simulink model "click_transpose"  (Simulink 10.0)
settings: Solver=VariableStepAuto  StartTime=0.0  StopTime=4  RelTol=1e-3
undefined symbols (not defined in the file or in its folder): DiscIntNeverNeededParam, q0, Tc
settings Model: LogicAnalyzerSignalOrdering=de64767a-5a6d-4200-a971-f55b6b3f8a08  Creator=swl782203812  LastModifiedBy=swl782203812
settings DataIOCC: SaveFormat=Dataset  ReturnWorkspaceOutputs=on
settings OptimizationCC: LifeSpan=auto
settings DebuggingCC: UnderspecifiedInitializationDetection=Simplified  MergeDetectMultiDrivingBlocksExec=error  SFUnexpectedBacktrackingDiag=error  SFNoUnconditionalDefaultTransitionDiag=error  SFExecutionAtInitializationDiag=warning
settings HardwareCC: ProdBitPerPointer=64  ProdBitPerSizeT=64  ProdBitPerPtrDiffT=64  ProdLargestAtomicFloat=Float  ProdIntDivRoundTo=Zero  ProdEndianess=LittleEndian  ProdWordSize=64  ProdHWDeviceType=Intel->x86-64 (Windows64)
settings ModelReferenceCC: PropagateSignalLabelsOutOfModel=on
settings SFSimCC: SimUseLocalCustomCode=on
settings RTWCC: RTWUseLocalCustomCode=on
settings CodeAppCC: StateflowObjectComments=off
settings GRTTargetCC: TargetLangStandard=C99 (ISO)  CombineOutputUpdateFcns=on  GRTInterface=off
settings ConfigComp: CovMetricSettings=dwe  CovHtmlReporting=off  CovSaveCumulativeToWorkspaceVar=off  CovSaveSingleToWorkspaceVar=off

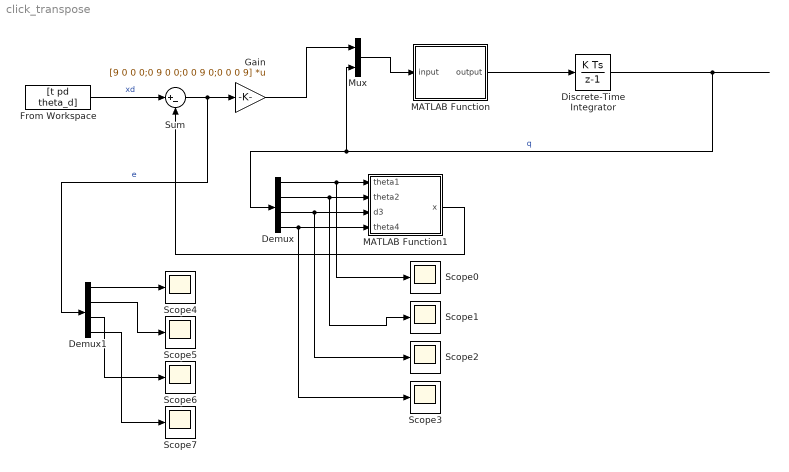
== system click_transpose ==
  Demux : Demux
  Demux1 : Demux
  Discrete-Time Integrator : DiscreteIntegrator  InitialCondition=q0  SampleTime=Tc  ICPrevOutput=DiscIntNeverNeededParam  ICPrevScaledInput=DiscIntNeverNeededParam
  From Workspace : FromWorkspace  VariableName=[t pd theta_d]  SampleTime=Tc
  Gain : Gain  Gain=[9 0 0 0;0 9 0 0;0 0 9 0;0 0 0 9]  Multiplication=Matrix(K*u) (u vector)
  MATLAB Function : MATLAB Function  TreatAsAtomicUnit=on
  MATLAB Function1 : MATLAB Function  TreatAsAtomicUnit=on
  Mux : Mux  Inputs=2
  Scope{0..7} (8 alike) : Scope
  Sum : Sum  Inputs=|+-
  wires:
  From Workspace/1 -> Sum/1  "xd"
  Sum/1 -> Demux1/1, Gain/1  "e"
  Discrete-Time Integrator/1 -> Mux/2, Demux/1  "q"
  Gain/1 -> Mux/1
  MATLAB Function1/1(x) -> Sum/2
  Demux/1 -> Scope0/1, MATLAB Function1/1(theta1)
  Demux/2 -> Scope1/1, MATLAB Function1/2(theta2)
  Demux/3 -> Scope2/1, MATLAB Function1/3(d3)
  Demux/4 -> Scope3/1, MATLAB Function1/4(theta4)
  MATLAB Function/1(output) -> Discrete-Time Integrator/1
  Mux/1 -> MATLAB Function/1(input)
  Demux1/1 -> Scope4/1
  Demux1/2 -> Scope5/1
  Demux1/3 -> Scope6/1
  Demux1/4 -> Scope7/1

== matlab function MATLAB Function ==
  data: input input double; output output double
function output=Jacobian_tranpose(input)
%INPUT is (theta1, theta2, d3, theta4,xd_dot_plus_Ke) 
theta1=input(5,:); d1=0; a1=0.5; alpha1=0; %parameter link1
theta2=input(6,:); d2=0; a2=0.5; alpha2=0; %parameter link2
theta3=0; d3=input(7,:); a3=0; alpha3=0;  %parameter link3
theta4=input(8,:); d4=0; a4=0; alpha4=0;  %parameter link4
 T01=DHmatrix(theta1,d1,a1,alpha1);
 T12=DHmatrix(theta2,d2,a2,alpha2);
 T23=DHmatrix(theta3,d3,a3,alpha3);
 T34=DHmatrix(theta4,d4,a4,alpha4);
 T02=T01*T12;
 T03=T01*T12*T23;
 T04=T01*T12*T23*T34;
P0=[0;0;0];
P1=T01(1:3,4);
P3=T03(1:3,4);
P4=T04(1:3,4);

Z0=[0;0;1];
Jv1=cross(Z0,(P4-P0));
Jv2=cross(Z0,(P4-P1));
Jv3=Z0;
Jv4=cross(Z0,(P4-P3));
Jv=[Jv1 Jv2 Jv3 Jv4;1 1 0 1];
output=Jv'*input(1:4,:);
end

function [Mdh] = DHmatrix(theta,d,a,alpha)
%DHMATRIX Summary of this function goes here
%   inputannya DH parameter
Mdh=[cos(theta) -sin(theta)*cos(alpha) sin(theta)*sin(alpha) a*cos(theta);
     sin(theta) cos(theta)*cos(alpha)  -cos(theta)*sin(alpha) a*sin(theta);
     0,sin(alpha),cos(alpha),d;
     0,0,0,1];
end

== matlab function MATLAB Function1 ==
  data: x output double; theta1 input double; theta2 input double; d3 input double; theta4 input double
function x = direct_kinematic(theta1,theta2,d3,theta4)
     d1=0; a1=0.5; alpha1=0; %parameter link1
     d2=0; a2=0.5; alpha2=0; %parameter link2
theta3=0;  a3=0; alpha3=0;  %parameter link3
     d4=0; a4=0; alpha4=0;  %parameter link4
 T01=DHmatrix(theta1,d1,a1,alpha1);
 T12=DHmatrix(theta2,d2,a2,alpha2);
 T23=DHmatrix(theta3,d3,a3,alpha3);
 T34=DHmatrix(theta4,d4,a4,alpha4);
 T04=T01*T12*T23*T34;
 theta_prime=theta1+theta2+theta4;
x=[T04(1:3,4);theta_prime];
end

function [Mdh] = DHmatrix(theta,d,a,alpha)
%DHMATRIX Summary of this function goes here
%   inputannya DH parameter
Mdh=[cos(theta) -sin(theta)*cos(alpha) sin(theta)*sin(alpha) a*cos(theta);
     sin(theta) cos(theta)*cos(alpha)  -cos(theta)*sin(alpha) a*sin(theta);
     0,sin(alpha),cos(alpha),d;
     0,0,0,1];
end
